simulink model "CM620C_MotAg0Meas"  (R2013b)
settings: Solver=FixedStepDiscrete  SolverMode=SingleTasking  StartTime=0.0  StopTime=1  FixedStep=0.0000625  RelTol=1e-3
values from neighbouring files (symbols this model uses):
  ARCHGLBPRM_2PI_ULS_F32 = DataDict.Constant    [CM620C_MotAg0Meas_DataDict.m]
  COEFFTBLELMSIZE_CNT_U08 = DataDict.Constant    [CM620C_MotAg0Meas_DataDict.m]
  COEFFTBLSIZE_CNT_U08 = DataDict.Constant    [CM620C_MotAg0Meas_DataDict.m]
  CORRNTBLAGSTEPSIZE_MATRAD_F32 = DataDict.Constant    [CM620C_MotAg0Meas_DataDict.m]
  CORRNTBLSIDXOFFS_CNT_U16 = DataDict.Constant    [CM620C_MotAg0Meas_DataDict.m]
  CORRNTBLSIZE_CNT_U16 = DataDict.Constant    [CM620C_MotAg0Meas_DataDict.m]
  CORRNTBLSIZEMASK_CNT_U08 = DataDict.Constant    [CM620C_MotAg0Meas_DataDict.m]
  MOTAG0ERRTHD_MOTREV_U0P16 = DataDict.Constant    [CM620C_MotAg0Meas_DataDict.m]
  MotAg0PrtclFlt = DataDict.NTC    [CM620C_MotAg0Meas_DataDict.m]
  MOTAG0PRTCLFLTFAILSTEP_CNT_U16 = DataDict.Constant    [CM620C_MotAg0Meas_DataDict.m]
  MOTAG0PRTCLFLTPASSSTEP_CNT_U16 = DataDict.Constant    [CM620C_MotAg0Meas_DataDict.m]
  MOTAGCPTLIMFLTMASK_CNT_U32 = DataDict.Constant    [CM620C_MotAg0Meas_DataDict.m]
  MOTAGDELTAPERCORRNPT_CNT_U16 = DataDict.Constant    [CM620C_MotAg0Meas_DataDict.m]
  MOTAGFLTMASK_CNT_U32 = DataDict.Constant    [CM620C_MotAg0Meas_DataDict.m]
  MOTAGIDXMASK_CNT_U16 = DataDict.Constant    [CM620C_MotAg0Meas_DataDict.m]
  MOTAGLIMMASK_CNT_S32 = DataDict.Constant    [CM620C_MotAg0Meas_DataDict.m]
  MOTAGMGNLIMFLTMASK_CNT_U32 = DataDict.Constant    [CM620C_MotAg0Meas_DataDict.m]
  MOTAGMINWAITPERD_CNT_U32 = DataDict.Constant    [CM620C_MotAg0Meas_DataDict.m]
  MOTAGOFFS_CNT_S32 = DataDict.Constant    [CM620C_MotAg0Meas_DataDict.m]
  MOTAGOVFFLTMASK_CNT_U32 = DataDict.Constant    [CM620C_MotAg0Meas_DataDict.m]
  MOTAGSPITRSMMASK_CNT_U32 = DataDict.Constant    [CM620C_MotAg0Meas_DataDict.m]
  MOTAGVLTGFLTMASK_CNT_U32 = DataDict.Constant    [CM620C_MotAg0Meas_DataDict.m]
  NOMOTAGFLTMASK_CNT_U32 = DataDict.Constant    [CM620C_MotAg0Meas_DataDict.m]
  READBUFADR_CNT_U32 = DataDict.Constant    [CM620C_MotAg0Meas_DataDict.m]
  READBUFIDX_CNT_U08 = DataDict.Constant    [CM620C_MotAg0Meas_DataDict.m]
  SNSRAGMASK_CNT_U32 = DataDict.Constant    [CM620C_MotAg0Meas_DataDict.m]
  SNSRCNTMASK_CNT_U32 = DataDict.Constant    [CM620C_MotAg0Meas_DataDict.m]
  SPIAGCNTREGIDX_CNT_U08 = DataDict.Constant    [CM620C_MotAg0Meas_DataDict.m]
  SPIAGREGIDX_CNT_U08 = DataDict.Constant    [CM620C_MotAg0Meas_DataDict.m]
  SPISTATREGIDX_CNT_U08 = DataDict.Constant    [CM620C_MotAg0Meas_DataDict.m]
  SPITURNCNTRREGIDX_CNT_U08 = DataDict.Constant    [CM620C_MotAg0Meas_DataDict.m]
  STRTPTRINITVAL_CNT_U32 = DataDict.Constant    [CM620C_MotAg0Meas_DataDict.m]
  STRTPTRPERVAL_CNT_U32 = DataDict.Constant    [CM620C_MotAg0Meas_DataDict.m]
  TURNCNTRHALFOFFS_CNT_S16 = DataDict.Constant    [CM620C_MotAg0Meas_DataDict.m]
  TURNCNTROFFS_CNT_S16 = DataDict.Constant    [CM620C_MotAg0Meas_DataDict.m]
  TURNCNTRREGMASK_CNT_U32 = DataDict.Constant    [CM620C_MotAg0Meas_DataDict.m]
  VLDMOTAGFLTMASK_CNT_U32 = DataDict.Constant    [CM620C_MotAg0Meas_DataDict.m]
undefined symbols (not defined in the file or in its folder): NtcSts1, sigbuilder_block
libraries: simulink x41, FloatToFixd x1, NxtrMax x1
(part 7 of 7)

== stateflow chart CM620C_MotAg0Meas/MotAg0Meas/MotAg0MeasPer2/MotAg0Calcn/MotAg0Processing/Diagnostics/ Qualifier Sts/SetNtcSts/ISO Fault Debounce Design ==
  note: NTCSTS_PASSD           (0)
      | NTCSTS_FAILD             (1)
      | NTCSTS_PREPASSD   (2)
      | NTCSTS_PREFAILD     (3)
      |
      | SIGQLFR_NORES        (0)
      | SIGQLFR_PASSD         (1)
      | SIGQLFR_FAILD           (2)
  note: Pass Loop
  note: Fail Loop
  note: 
  (default) -> (junction 89)
  (junction 89) -> (junction 95) [order 1] : [NtcSts ==3]
  (junction 89) -> (junction 93) [order 2] : [NtcSts ==2]
  (junction 89) -> (junction 141) [order 3] : [NtcSts ==1]
      | { ErrAcc = 32767;
      | Qualifier =2;
      |  }
  (junction 89) -> (junction 141) [order 4] : [NtcSts ==0]
      | { ErrAcc = -32768;
      | Qualifier=1;
      | }
  (junction 95) -> (junction 103) [order 2]
  (junction 95) -> (junction 111) [order 1] : [ErrAcc <=0]
      | {ErrAcc = DebStep;}
  (junction 93) -> (junction 123) [order 2] : {
      | ErrAcc = ErrAcc - DebStep;
      | }
  (junction 93) -> (junction 123) [order 1] : [(ErrAcc - DebStep) <= -32768]
      | { ErrAcc = -32768;
      | Qualifier=1;
      | }
  (junction 103) -> (junction 111) [order 1] : [(ErrAcc + DebStep) <32767]
      | {ErrAcc = ErrAcc + DebStep;}
  (junction 103) -> (junction 111) [order 2] : {ErrAcc = 32767;
      | Qualifier =2;}
  (junction 123) -> (junction 141)
  (junction 111) -> (junction 141)
  (junction 141) -> (junction 159) [order 2] : {ErrAcc = 0;
      | Qualifier =0;
      | }
  (junction 141) -> (junction 159) [order 1] : [SvcClr ==0]
  data: NtcSts input uint8; Qualifier output uint8; DebStep input uint16; ErrAcc local int16; SvcClr input

== matlab function CM620C_MotAg0Meas/MotAg0Meas/MotAg0MeasInit1/Compute Correction Table/NVM Ok/Calculate Correction Table/Build Wave/Reconstructed Waveform Processing/Harmonic Coefficient Processing/SinCos (Use library function from NxtrMath)/Truth Table ==
  data: RngLimitedSin input; RngLimitedCos input; ThetaIndex input; Sin output; Cos output; SIN225DEG_ULS_F32 input; SIN675DEG_ULS_F32 input; SIN450DEG_ULS_F32 input
function [Sin, Cos] = fcn(RngLimitedSin, RngLimitedCos, ThetaIndex, SIN225DEG_ULS_F32, SIN675DEG_ULS_F32, SIN450DEG_ULS_F32)

aVarTruthTableCondition_1 = false;
aVarTruthTableCondition_2 = false;
aVarTruthTableCondition_3 = false;
aVarTruthTableCondition_4 = false;
aVarTruthTableCondition_5 = false;
aVarTruthTableCondition_6 = false;
aVarTruthTableCondition_7 = false;
aVarTruthTableCondition_8 = false;
aVarTruthTableCondition_9 = false;
aVarTruthTableCondition_10 = false;
aVarTruthTableCondition_11 = false;
aVarTruthTableCondition_12 = false;
aVarTruthTableCondition_13 = false;
aVarTruthTableCondition_14 = false;
aVarTruthTableCondition_15 = false;
aVarTruthTableCondition_16 = false;


% 0      <= Theta < 11.25 &&
% 348.75 <= Theta < 360

aVarTruthTableCondition_1 = logical(ThetaIndex == 0);

% 11.25  <= Theta < 33.75

aVarTruthTableCondition_2 = logical(ThetaIndex == 1);

% 33.75  <= Theta < 56.25

aVarTruthTableCondition_3 = logical(ThetaIndex == 2);

% 56.25  <= Theta < 78.75

aVarTruthTableCondition_4 = logical(ThetaIndex == 3);

% 78.75  <= Theta < 101.25

aVarTruthTableCondition_5 = logical(ThetaIndex == 4);

% 101.25 <= Theta < 123.75

aVarTruthTableCondition_6 = logical(ThetaIndex == 5);

% 123.75 <= Theta < 146.25

aVarTruthTableCondition_7 = logical(ThetaIndex == 6);

% 146.25 <= Theta < 168.75

aVarTruthTableCondition_8 = logical(ThetaIndex == 7);

% 168.75 <= Theta < 191.25

aVarTruthTableCondition_9 = logical(ThetaIndex == 8);

% 191.25 <= Theta < 213.75

aVarTruthTableCondition_10 = logical(ThetaIndex == 9);

% 213.75 <= Theta < 236.25

aVarTruthTableCondition_11 = logical(ThetaIndex == 10);

% 236.25 <= Theta < 258.75

aVarTruthTableCondition_12 = logical(ThetaIndex == 11);

% 258.75 <= Theta < 281.25

aVarTruthTableCondition_13 = logical(ThetaIndex == 12);

% 281.25 <= Theta < 303.75

aVarTruthTableCondition_14 = logical(ThetaIndex == 13);

% 303.75 <= Theta < 326.75

aVarTruthTableCondition_15 = logical(ThetaIndex == 14);

% 326.75 <= Theta < 348.75

aVarTruthTableCondition_16 = logical(ThetaIndex == 15);

if (aVarTruthTableCondition_1)
    aFcnTruthTableAction_1();
elseif (aVarTruthTableCondition_2)
    aFcnTruthTableAction_2();
elseif (aVarTruthTableCondition_3)
    aFcnTruthTableAction_3();
elseif (aVarTruthTableCondition_4)
    aFcnTruthTableAction_4();
elseif (aVarTruthTableCondition_5)
    aFcnTruthTableAction_5();
elseif (aVarTruthTableCondition_6)
    aFcnTruthTableAction_6();
elseif (aVarTruthTableCondition_7)
    aFcnTruthTableAction_7();
elseif (aVarTruthTableCondition_8)
    aFcnTruthTableAction_8();
elseif (aVarTruthTableCondition_9)
    aFcnTruthTableAction_9();
elseif (aVarTruthTableCondition_10)
    aFcnTruthTableAction_10();
elseif (aVarTruthTableCondition_11)
    aFcnTruthTableAction_11();
elseif (aVarTruthTableCondition_12)
    aFcnTruthTableAction_12();
elseif (aVarTruthTableCondition_13)
    aFcnTruthTableAction_13();
elseif (aVarTruthTableCondition_14)
    aFcnTruthTableAction_14();
elseif (aVarTruthTableCondition_15)
    aFcnTruthTableAction_15();
else % Default
    aFcnTruthTableAction_16();
end

function aFcnTruthTableAction_1()

% Example action 1 called from D1 & D2 column in condition table

Sin = RngLimitedSin;
Cos = RngLimitedCos;

function aFcnTruthTableAction_2()


Sin =  SIN675DEG_ULS_F32 * RngLimitedSin + SIN225DEG_ULS_F32 * RngLimitedCos;
Cos = -SIN225DEG_ULS_F32 * RngLimitedSin + SIN675DEG_ULS_F32 * RngLimitedCos;

function aFcnTruthTableAction_3()


Sin =  SIN450DEG_ULS_F32 * RngLimitedSin + SIN450DEG_ULS_F32 * RngLimitedCos;
Cos = -SIN450DEG_ULS_F32 * RngLimitedSin + SIN450DEG_ULS_F32 * RngLimitedCos;

function aFcnTruthTableAction_4()


Sin =  SIN225DEG_ULS_F32 * RngLimitedSin + SIN675DEG_ULS_F32 * RngLimitedCos;
Cos = -SIN675DEG_ULS_F32 * RngLimitedSin + SIN225DEG_ULS_F32 * RngLimitedCos;

function aFcnTruthTableAction_5()


Sin = RngLimitedCos;
Cos = -RngLimitedSin;

function aFcnTruthTableAction_6()


Sin = -SIN225DEG_ULS_F32 * RngLimitedSin + SIN675DEG_ULS_F32 * RngLimitedCos;
Cos = -SIN675DEG_ULS_F32 * RngLimitedSin + -SIN225DEG_ULS_F32 * RngLimitedCos;

function aFcnTruthTableAction_7()


Sin = -SIN450DEG_ULS_F32 * RngLimitedSin + SIN450DEG_ULS_F32 * RngLimitedCos;
Cos = -SIN450DEG_ULS_F32 * RngLimitedSin + -SIN450DEG_ULS_F32 * RngLimitedCos;

function aFcnTruthTableAction_8()


Sin = -SIN675DEG_ULS_F32 * RngLimitedSin + SIN225DEG_ULS_F32 * RngLimitedCos;
Cos = -SIN225DEG_ULS_F32 * RngLimitedSin + -SIN675DEG_ULS_F32 * RngLimitedCos;

function aFcnTruthTableAction_9()


Sin = -RngLimitedSin;
Cos = -RngLimitedCos;

function aFcnTruthTableAction_10()


Sin = -SIN675DEG_ULS_F32 * RngLimitedSin + -SIN225DEG_ULS_F32 * RngLimitedCos;
Cos =  SIN225DEG_ULS_F32 * RngLimitedSin + -SIN675DEG_ULS_F32 * RngLimitedCos;

function aFcnTruthTableAction_11()


Sin = -SIN450DEG_ULS_F32 * RngLimitedSin + -SIN450DEG_ULS_F32 * RngLimitedCos;
Cos =  SIN450DEG_ULS_F32 * RngLimitedSin + -SIN450DEG_ULS_F32 * RngLimitedCos;

function aFcnTruthTableAction_12()


Sin = -SIN225DEG_ULS_F32 * RngLimitedSin + -SIN675DEG_ULS_F32 * RngLimitedCos;
Cos =  SIN675DEG_ULS_F32 * RngLimitedSin + -SIN225DEG_ULS_F32 * RngLimitedCos;

function aFcnTruthTableAction_13()


Sin = -RngLimitedCos;
Cos =  RngLimitedSin;

function aFcnTruthTableAction_14()


Sin =  SIN225DEG_ULS_F32 * RngLimitedSin + -SIN675DEG_ULS_F32 * RngLimitedCos;
Cos =  SIN675DEG_ULS_F32 * RngLimitedSin +  SIN225DEG_ULS_F32 * RngLimitedCos;

function aFcnTruthTableAction_15()


Sin =  SIN450DEG_ULS_F32 * RngLimitedSin + -SIN450DEG_ULS_F32 * RngLimitedCos;
Cos =  SIN450DEG_ULS_F32 * RngLimitedSin +  SIN450DEG_ULS_F32 * RngLimitedCos;

function aFcnTruthTableAction_16()

% Example action 2 called from D3 column in condition table

Sin =  SIN675DEG_ULS_F32 * RngLimitedSin + -SIN225DEG_ULS_F32 * RngLimitedCos;
Cos =  SIN225DEG_ULS_F32 * RngLimitedSin +  SIN675DEG_ULS_F32 * RngLimitedCos;

== matlab function CM620C_MotAg0Meas/MotAg0Meas/MotAg0MeasInit1/Compute Correction Table/NVM Ok/Calculate Correction Table/Change Correction Coordinate/Waveform Coordinate Change/Calculate Index Scale/Truth Table ==
  data: ReconWfrm_0 input; IndexScale output single; LoopIndex input; ARCHGLBPRM_2PI_ULS_F32 input
function IndexScale = fcn(ReconWfrm_0, LoopIndex, ARCHGLBPRM_2PI_ULS_F32)

aVarTruthTableCondition_1 = false;
aVarTruthTableCondition_2 = false;
aVarTruthTableCondition_3 = false;


% First entry in reconstructed waveform is >= 0

aVarTruthTableCondition_1 = logical(ReconWfrm_0 >= 0);

% Reconstructed waveform is positively wrapped around

aVarTruthTableCondition_2 = logical(ReconWfrm_0 > LoopIndex);

% Reconstructed waveform is negatively wrapped around

aVarTruthTableCondition_3 = logical((ReconWfrm_0 + ARCHGLBPRM_2PI_ULS_F32) <= LoopIndex);

if (aVarTruthTableCondition_1 && aVarTruthTableCondition_2)
    aFcnTruthTableAction_1();
elseif (aVarTruthTableCondition_1)
    aFcnTruthTableAction_3();
elseif (aVarTruthTableCondition_3)
    aFcnTruthTableAction_2();
else % Default
    aFcnTruthTableAction_3();
end

function aFcnTruthTableAction_1()

% Reconstructed waveform is positively wrapped around - add 2pi for alignment

IndexScale = LoopIndex + ARCHGLBPRM_2PI_ULS_F32;

function aFcnTruthTableAction_2()

% Reconstructed waveform is negatively wrapped around - subtract 2pi for alignment

IndexScale = LoopIndex - ARCHGLBPRM_2PI_ULS_F32;

function aFcnTruthTableAction_3()

% Reconstructed waveform and loop index are not wrapped relative to one another

IndexScale = LoopIndex;
